simulink model "a0_px4demo_PositionAndRateController"  (R2023b)
settings: Solver=FixedStepAuto  StartTime=0.0  StopTime=inf  RelTol=1e-3  EnableMultiTasking=on
PreLoadFcn:
  | if ispc
  | SampleTime = 0.01
  | PID_x_P = 0.8580043859649122
  | PID_x_I = 0
  | PID_x_D = 0.3097345132743363
  | PID_x_N = 10
  | 
  | PID_vx_P = 9.961622807017545
  | PID_vx_I = 0
  | PID_vx_D = 0.1081612586037365
  | PID_vx_N = 10
  | 
  | PID_y_P = 0.85
  | PID_y_I = 0
  | PID_y_D = 0.3
  | PID_y_N = 10
  | 
  | PID_vy_P = 10
  | PID_vy_I = 0
  | PID_vy_D = 0.1
  | PID_vy_N = 10
  | 
  | PID_z_P = 2.001693480101609
  | PID_z_I = 0.1
  | PID_z_D = 0.5
  | PID_z_N = 10
  | 
  | PID_vz_P = 1.906858594411516
  | PID_vz_I = 0.1
  | PID_vz_D = 0.09829059829059829
  | PID_vz_N = 10
  | 
  | PID_yaw_P = 0.08024000000000001
  | PID_yaw_I = 0.005
  | PID_yaw_D = 0.075
  | PID_yaw_N = 100
  | 
  | elseif isunix
  | SampleTime = 0.004
  | PID_x_P = 0.6
  | PID_x_I = 0
  | PID_x_D = 0.15
  | PID_x_N = 1
  | 
  | PID_vx_P = 8
  | PID_vx_I = 0
  | PID_vx_D = 0.05
  | PID_vx_N = 1
  | 
  | PID_y_P = 0.6
  | PID_y_I = 0
  | PID_y_D = 0.15
  | PID_y_N = 1
  | 
  | PID_vy_P = 8
  | PID_vy_I = 0
  | PID_vy_D = 0.05
  | PID_vy_N = 1
  | 
  | PID_z_P = 1.5
  | ... (+15 lines)
undefined symbols (not defined in the file or in its folder): dev, Main, pwm_output0
libraries: slpidlib x9, px4uORBlib x4, simulink_extras x3, sharedtransform x1, px4lib x1, sharedTrackingLibrary x1
(part 2 of 2)

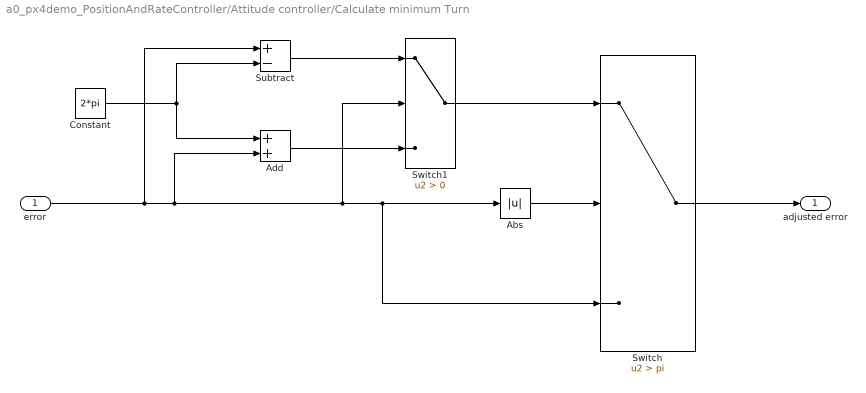
== system a0_px4demo_PositionAndRateController/Attitude controller/Calculate minimum Turn ==
  error : Inport
  Abs : Abs  SaturateOnIntegerOverflow=off
  Add : Sum
  Constant : Constant  Value=2*pi  SampleTime=-1
  Subtract : Sum  Inputs=+-
  Switch : Switch  Criteria=u2 > Threshold  Threshold=pi  SaturateOnIntegerOverflow=off  InputSameDT=off
  Switch1 : Switch  Criteria=u2 > Threshold  SaturateOnIntegerOverflow=off  InputSameDT=off
  adjusted error : Outport
  wires:
  Switch/1 -> adjusted error/1
  Abs/1 -> Switch/2
  Constant/1 -> Subtract/2, Add/1
  Subtract/1 -> Switch1/1
  Add/1 -> Switch1/3
  error/1 -> Subtract/1, Switch/3, Abs/1, Switch1/2, Add/2
  Switch1/1 -> Switch/1

== matlab function a0_px4demo_PositionAndRateController/Position & Altitude controller/Rotation mat  ==
  data: theta input; R output
function R = fcn(theta)
R = [cos(theta) -sin(theta); sin(theta) cos(theta)]';

== matlab function a0_px4demo_PositionAndRateController/Generate Residual/MATLAB Function - Generate Predicted Output ==
  data: state_Estimated input; phi_Predicted output; u2 input; u3 input; u4 input; theta_Predicted output; psi_Predicted output
function [phi_Predicted,theta_Predicted,psi_Predicted] = generatePredictedOutput(state_Estimated,u2,u3,u4)

%   Copyright 2017 The MathWorks, Inc.

%#codegen

% Given state estimates at previous time (k-1) utilizing measurements up to
% (k-1), predict states at current step.
state_Predicted = uavStateFcn(state_Estimated,u2,u3,u4); % xhat[k|k-1]
% Generate output estimate, again without utilizing the measurement at
% current time.
phi_Predicted = uavMeasurementFcn1(state_Predicted); % y[k|k-1]
theta_Predicted = uavMeasurementFcn2(state_Predicted); % y[k|k-1]
psi_Predicted = uavMeasurementFcn3(state_Predicted); % y[k|k-1]
end

== matlab function a0_px4demo_PositionAndRateController/Simulink Function/uavstate ==
  data: x input; x output; u2 input; u3 input; u4 input
function x = uavStateFcn_simulink(x,u2,u3,u4)

% Euler integration of continuous-time dynamics x'=f(x) with sample time dt
dt = 0.01; % [s] Sample time
x = x + vdpStateFcnContinuous(x,u2,u3,u4)*dt;
end

function dxdt = vdpStateFcnContinuous(x,u2,u3,u4)
%Ix=x(10);Iy=x(12);Iz=x(14);K1=x(16);K2=x(16);
dxdt = [x(2); x(3); (x(12)-x(14))/x(10)*x(6)*x(9) + x(16)*u2/x(10);...
        x(5); x(6); (x(14)-x(10))/x(12)*x(3)*x(9) + x(16)*u3/x(12);...
        x(8); x(9); (x(10)-x(12))/x(14)*x(3)*x(6) + x(18)*u4/x(14);...
        x(11);0;x(13);0;x(15);0;x(17);0;x(19);0;];
end
